simulink model "problem2"  (R2020b)
settings: Solver=VariableStepAuto  StartTime=0.0  StopTime=100  RelTol=1e-3
undefined symbols (not defined in the file): b, K1, K2, m1, m2
settings Model: Creator=Hp  LastModifiedBy=Hp

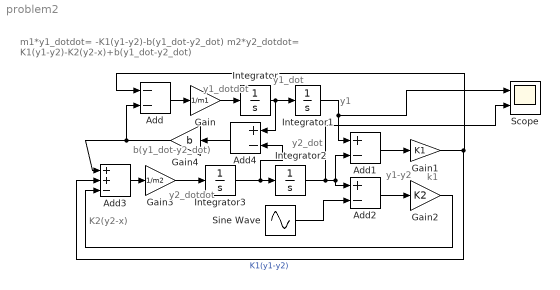
== system problem2 ==
  note: K2(y2-x)
  note: y1-y2
  note: y2_dot
  note: y2_dotdot
  note: b(y1_dot-y2_dot)
  note: k1
  note: y1
  note: y1_dot
  note: y1_dotdot
  note: m1*y1_dotdot= -K1(y1-y2)-b(y1_dot-y2_dot)
      |
      | m2*y2_dotdot= K1(y1-y2)-K2(y2-x)+b(y1_dot-y2_dot)
  Add : Sum  Inputs=--
  Add1 : Sum  Inputs=+-
  Add2 : Sum  Inputs=+-
  Add3 : Sum  Inputs=++-
  Add4 : Sum  Inputs=+-
  Gain : Gain  Gain=1/m1
  Gain1 : Gain  Gain=K1
  Gain2 : Gain  Gain=K2
  Gain3 : Gain  Gain=1/m2
  Gain4 : Gain  Gain=b
  Integrator{,1..3} (4 alike) : Integrator
  Scope : Scope  NumInputPorts=2
  Sine Wave : Sin  SampleTime=0
  wires:
  Gain/1 -> Integrator/1
  Integrator/1 -> Add4/1, Integrator1/1
  Add/1 -> Gain/1
  Add2/1 -> Gain2/1
  Add3/1 -> Gain3/1
  Add1/1 -> Gain1/1
  Integrator1/1 -> Scope/1, Add1/1
  Integrator2/1 -> Scope/2, Add2/1, Add1/2
  Sine Wave/1 -> Add2/2
  Integrator3/1 -> Add4/2, Integrator2/1
  Gain3/1 -> Integrator3/1
  Gain4/1 -> Add/2, Add3/1
  Gain1/1 -> Add3/2, Add/1  "K1(y1-y2)"
  Gain2/1 -> Add3/3
  Add4/1 -> Gain4/1
